simulink model "Test_N3"  (R2020b)
settings: Solver=ode3  StartTime=0.0  StopTime=inf  FixedStep=0.05  RelTol=1e-3
libraries: XBotBlockToolbox x4, Utilities x3, Sensors x2

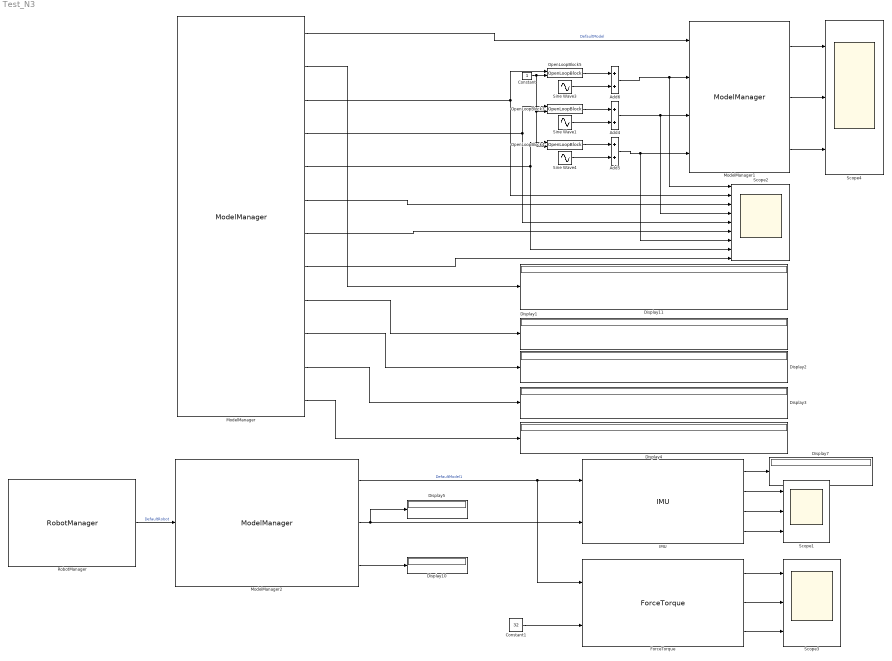
== system Test_N3 ==
  Add4 : Sum
  Add5 : Sum
  Add6 : Sum
  Constant : Constant
  Constant1 : Constant  Value=32
  Display{1..5,7,10..11} (8 alike) : Display
  ForceTorque : Sensors/ForceTorque  ManagerName=DefaultModel1  ManagerType=Model  ForceTorqueList={ 'f', 't', 'w' }
  IMU : Sensors/IMU  ManagerName=DefaultModel1  ManagerType=Model  IMUList={ 'orient', 'quat', 'a', 'omega' }
  ModelManager : XBotBlockToolbox/ModelManager  ModelName=DefaultModel  RobotName=DefaultRobot  UseExtModel=Off  SyncWithRobot=Off  GetFloatingBaseList={}  SetFloatingBaseComponent=Off  GravityRequest=Off  ReadingsList={ 'q_ID', 'qJ', 'qJdot', 'tau', 'qJ_ref', 'qJdot_ref', 'tau_ref' }  MechanicalLimitsList={ 'q_min', 'q_max', 'qdot_max', 'tau_max' }  MechanicalLimitsCheck=Off  MechanicalLimitsEnforce=Off  SensorList={}  ReferencesList={}  OldModelName=DefaultModel
  ModelManager1 : XBotBlockToolbox/ModelManager  ModelName=DefaultModel  RobotName=DefaultRobot  UseExtModel=On  SyncWithRobot=Off  GetFloatingBaseList={}  SetFloatingBaseComponent=Off  GravityRequest=Off  ReadingsList={}  MechanicalLimitsList={}  MechanicalLimitsCheck=On  MechanicalLimitsEnforce=On  SensorList={}  ReferencesList={ 'qJ_ref', 'qJdot_ref', 'tau_ref' }  OldModelName=DefaultModel
  ModelManager2 : XBotBlockToolbox/ModelManager  ModelName=DefaultModel1  RobotName=DefaultRobot  UseExtModel=Off  SyncWithRobot=On  GetFloatingBaseList={}  SetFloatingBaseComponent=Off  GravityRequest=Off  ReadingsList={}  MechanicalLimitsList={}  MechanicalLimitsCheck=Off  MechanicalLimitsEnforce=Off  SensorList={ 'IMU', 'FT' }  ReferencesList={}  OldModelName=DefaultModel1
  OpenLoopBlock3 : Utilities/OpenLoopBlock  SystemSampleTime=-1  VariantActivationTime=update diagram  Latency=0  AutoFrameSizeCalculation=off
  OpenLoopBlock4 : Utilities/OpenLoopBlock  SystemSampleTime=-1  VariantActivationTime=update diagram  Latency=0  AutoFrameSizeCalculation=off
  OpenLoopBlock5 : Utilities/OpenLoopBlock  SystemSampleTime=-1  VariantActivationTime=update diagram  Latency=0  AutoFrameSizeCalculation=off
  RobotManager : XBotBlockToolbox/RobotManager  RobotName=DefaultRobot  ModelName=DefaultModel  UseExtRobot=Off  SyncWithModel=Off  ReadingsList={}  MechanicalLimitsList={}  MechanicalLimitsCheck=Off  MechanicalLimitsEnforce=Off  SensorList={}  ReferencesList={}  OldRobotName=DefaultRobot
  Scope1 : Scope  NumInputPorts=3
  Scope2 : Scope  NumInputPorts=9
  Scope3 : Scope  NumInputPorts=3
  Scope4 : Scope  NumInputPorts=3
  Sine Wave1 : Sin  Amplitude=20  SampleTime=0
  Sine Wave3 : Sin  Amplitude=0.2  SampleTime=0
  Sine Wave4 : Sin  Amplitude=300  SampleTime=0
  wires:
  Add4/1 -> ModelManager1/3, Scope2/4
  ModelManager/1 -> ModelManager1/1  "DefaultModel"
  Add5/1 -> ModelManager1/4, Scope2/7
  Add6/1 -> ModelManager1/2, Scope2/1
  ModelManager/4 -> OpenLoopBlock3/1, Scope2/5
  ModelManager/5 -> OpenLoopBlock4/1, Scope2/8
  Sine Wave4/1 -> Add5/2
  ModelManager/3 -> OpenLoopBlock5/1, Scope2/2
  OpenLoopBlock3/1 -> Add4/1
  ModelManager/7 -> Scope2/6
  ModelManager/6 -> Scope2/3
  OpenLoopBlock4/1 -> Add5/1
  Sine Wave3/1 -> Add6/2
  OpenLoopBlock5/1 -> Add6/1
  Sine Wave1/1 -> Add4/2
  ModelManager/8 -> Scope2/9
  ModelManager/9 -> Display1/1
  ModelManager/10 -> Display2/1
  ModelManager/11 -> Display3/1
  ModelManager/12 -> Display4/1
  Constant/1 -> OpenLoopBlock4/2, OpenLoopBlock3/2, OpenLoopBlock5/2
  ForceTorque/2 -> Scope3/2
  ForceTorque/1 -> Scope3/1
  IMU/1 -> Display7/1
  ModelManager2/2 -> IMU/2, Display5/1
  IMU/2 -> Scope1/1
  IMU/4 -> Scope1/3
  IMU/3 -> Scope1/2
  ForceTorque/3 -> Scope3/3
  ModelManager2/3 -> Display10/1
  ModelManager2/1 -> ForceTorque/1, IMU/1  "DefaultModel1"
  RobotManager/1 -> ModelManager2/1  "DefaultRobot"
  Constant1/1 -> ForceTorque/2
  ModelManager1/1 -> Scope4/1
  ModelManager1/2 -> Scope4/2
  ModelManager1/3 -> Scope4/3
  ModelManager/2 -> Display11/1
